simulink model "partexp"  (R2017a)
settings: Solver=VariableStepAuto  StartTime=0.0  StopTime=10.0  RelTol=1e-3
settings Model: Creator=adi  LastModifiedBy=adi

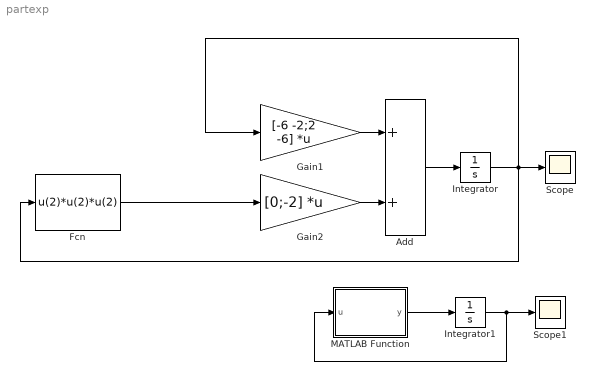
== system partexp ==
  Add : Sum
  Fcn : Fcn  Expr=u(2)*u(2)*u(2)
  Gain1 : Gain  Gain=[-6 -2;2 -6]  Multiplication=Matrix(K*u)
  Gain2 : Gain  Gain=[0;-2]  Multiplication=Matrix(K*u)
  Integrator : Integrator
  Integrator1 : Integrator  InitialCondition=[2;2]
  MATLAB Function : MATLAB Function  TreatAsAtomicUnit=on
  Scope : Scope
  Scope1 : Scope
  wires:
  Gain1/1 -> Add/1
  Gain2/1 -> Add/2
  Add/1 -> Integrator/1
  Integrator/1 -> Fcn/1, Gain1/1, Scope/1
  Fcn/1 -> Gain2/1
  MATLAB Function/1(y) -> Integrator1/1
  Integrator1/1 -> MATLAB Function/1(u), Scope1/1

== matlab function partexp/MATLAB Function ==
  data: u input; y output
function y = fcn(u)

y = [-6 2;2 -6]*u+[0;-2]*u(2)^3;
